simulink model "Proposed_converter"  (R2023b)
settings: Solver=VariableStepAuto  StartTime=0.0  StopTime=30e-3  RelTol=1e-3
undefined symbols (not defined in the file): pro
libraries: spsVoltageMeasurementLib x22, spsCurrentMeasurementLib x21, spsSeriesRLCBranchLib x17, spsDiodeLib x11, spsIdealSwitchLib x6, spsDCVoltageSourceLib x2, spspowerguiLib x2
settings Model: Creator=JesperBertelsen  LastModifiedBy=JesperBertelsen

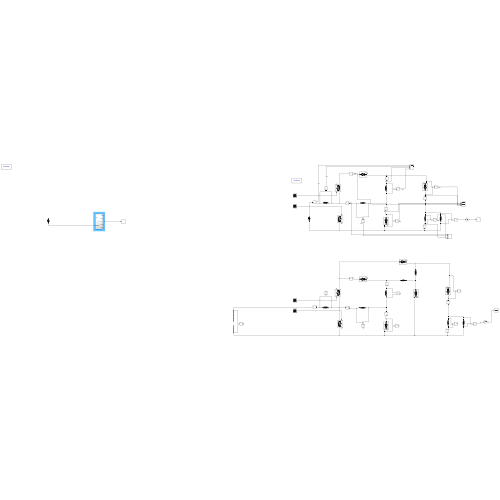
[thumbnail: Simulink's stored preview of the top-level diagram]
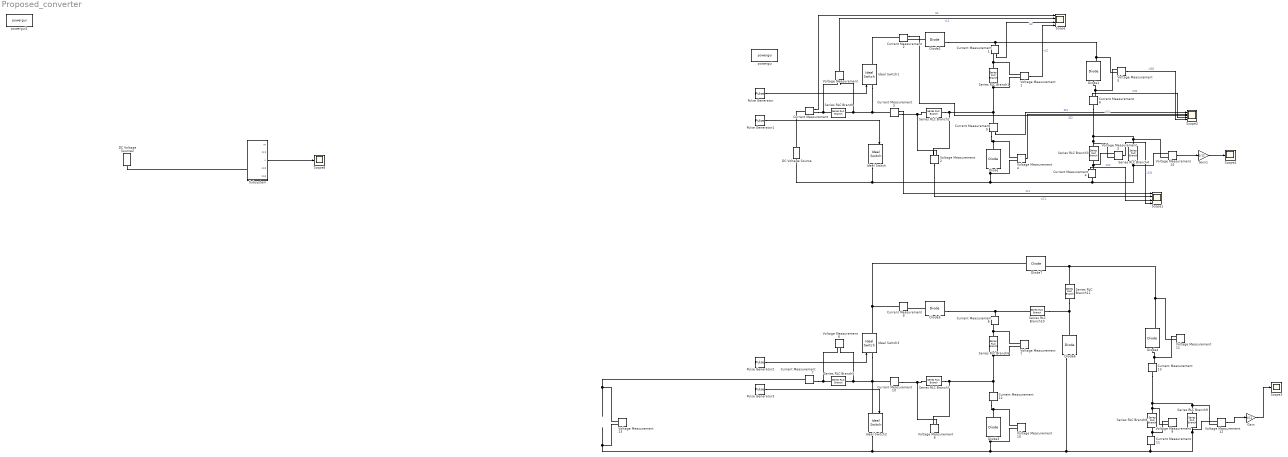
== system Proposed_converter ==
  Current Measurement{,1..13} (14 alike) : spsCurrentMeasurementLib/Current Measurement  PhasorSimulation=off  OutputType=Complex  PSBequivalent=0
  DC Voltage Source : spsDCVoltageSourceLib/DC Voltage Source  Amplitude=pro.Vi  Measurements=None
  DC Voltage Source2 : spsDCVoltageSourceLib/DC Voltage Source  Amplitude=pro.Vi  Measurements=None
  Diode{,1..7} (8 alike) : spsDiodeLib/Diode  Ron=pro.rD  Lon=0  Vf=0.8  IC=0  UseSnubber=0  Rs=0  Cs=0  Measurements=on
  Gain : Gain  Gain=1/12
  Gain1 : Gain  Gain=1/12
  Ideal Switch{,1..3} (4 alike) : spsIdealSwitchLib/Ideal Switch  Ron=0.001  Lon=0  IC=0  Rs=1e5  Cs=inf  Measurements=on
  Pulse Generator{,1..3} (4 alike) : DiscretePulseGenerator  PulseType=Time based  Period=1/pro.f  PulseWidth=50
  Scope : Scope  NumInputPorts=4
  Scope1 : Scope  NumInputPorts=4
  Scope2 : Scope  NumInputPorts=5
  Scope3 : Scope
  Scope4 : Scope
  Scope8 : Scope
  Series RLC Branch : spsSeriesRLCBranchLib/Series RLC Branch  LConnTagsString=__new0  RConnTagsString=__new0  BranchType=L  Resistance=1  Inductance=pro.L1  SetiL0=off  InitialCurrent=0  Capacitance=1e-6  Setx0=off  InitialVoltage=0  Measurements=Branch voltage and current
  Series RLC Branch1 : spsSeriesRLCBranchLib/Series RLC Branch  LConnTagsString=__new0  RConnTagsString=__new0  BranchType=L  Resistance=1  Inductance=pro.L2  SetiL0=off  InitialCurrent=0  Capacitance=1e-6  Setx0=off  InitialVoltage=0  Measurements=Branch voltage and current
  Series RLC Branch10 : spsSeriesRLCBranchLib/Series RLC Branch  LConnTagsString=__new0  RConnTagsString=__new0  BranchType=C  Resistance=1  Inductance=1e-3  SetiL0=off  InitialCurrent=0  Capacitance=pro.C1  Setx0=off  InitialVoltage=0  Measurements=Branch voltage and current
  Series RLC Branch11 : spsSeriesRLCBranchLib/Series RLC Branch  LConnTagsString=__new0  RConnTagsString=__new0  BranchType=L  Resistance=1  Inductance=pro.L2  SetiL0=off  InitialCurrent=0  Capacitance=1e-6  Setx0=off  InitialVoltage=0  Measurements=Branch voltage and current
  Series RLC Branch2 : spsSeriesRLCBranchLib/Series RLC Branch  LConnTagsString=__new0  RConnTagsString=__new0  BranchType=C  Resistance=1  Inductance=1e-3  SetiL0=off  InitialCurrent=0  Capacitance=pro.C1  Setx0=off  InitialVoltage=0  Measurements=Branch voltage and current
  Series RLC Branch3 : spsSeriesRLCBranchLib/Series RLC Branch  LConnTagsString=__new0  RConnTagsString=__new0  BranchType=C  Resistance=1  Inductance=1e-3  SetiL0=off  InitialCurrent=0  Capacitance=pro.C1  Setx0=off  InitialVoltage=0  Measurements=None
  Series RLC Branch4 : spsSeriesRLCBranchLib/Series RLC Branch  LConnTagsString=__new0  RConnTagsString=__new0  BranchType=R  Resistance=pro.R  Inductance=pro.L1  SetiL0=off  InitialCurrent=0  Capacitance=1e-6  Setx0=off  InitialVoltage=0  Measurements=None
  Series RLC Branch5 : spsSeriesRLCBranchLib/Series RLC Branch  LConnTagsString=__new0  RConnTagsString=__new0  BranchType=L  Resistance=1  Inductance=pro.L1  SetiL0=off  InitialCurrent=0  Capacitance=1e-6  Setx0=off  InitialVoltage=0  Measurements=Branch voltage and current
  Series RLC Branch6 : spsSeriesRLCBranchLib/Series RLC Branch  LConnTagsString=__new0  RConnTagsString=__new0  BranchType=L  Resistance=1  Inductance=pro.L2  SetiL0=off  InitialCurrent=0  Capacitance=1e-6  Setx0=off  InitialVoltage=0  Measurements=Branch voltage and current
  Series RLC Branch7 : spsSeriesRLCBranchLib/Series RLC Branch  LConnTagsString=__new0  RConnTagsString=__new0  BranchType=C  Resistance=1  Inductance=1e-3  SetiL0=off  InitialCurrent=0  Capacitance=pro.C1  Setx0=off  InitialVoltage=0  Measurements=Branch voltage and current
  Series RLC Branch8 : spsSeriesRLCBranchLib/Series RLC Branch  LConnTagsString=__new0  RConnTagsString=__new0  BranchType=C  Resistance=1  Inductance=1e-3  SetiL0=off  InitialCurrent=0  Capacitance=pro.C1  Setx0=off  InitialVoltage=0  Measurements=None
  Series RLC Branch9 : spsSeriesRLCBranchLib/Series RLC Branch  LConnTagsString=__new0  RConnTagsString=__new0  BranchType=R  Resistance=pro.R  Inductance=pro.L1  SetiL0=off  InitialCurrent=0  Capacitance=1e-6  Setx0=off  InitialVoltage=0  Measurements=None
  Subsystem : Subsystem
  Voltage Measurement{,1..14} (15 alike) : spsVoltageMeasurementLib/Voltage Measurement  PhasorSimulation=off  OutputType=Complex  PSBequivalent=0
  powergui : spspowerguiLib/powergui  Priority=1  SimulationMode=Continuous  SampleTime=50e-6  frequency=60  Iterations=50  frequencyindice=0  Pbase=100e6  ErrMax=1e-4  UnitsV=kV  UnitsW=MW  buscounter=0  FunctionMessages=off  echomessages=off  EnableUseOfTLC=off  CurrentSourceSwitches=off  DisableSnubberDevices=off  DisableRonSwitches=off  DisableVfSwitches=off  DisplayEquations=off  AutomaticDiscreteSolvers=off  SolverType=Tustin/Backward Euler (TBE)  Interpol=off  ExternalGateDelay=off  methode=off  Ts=100  x0status=blocks  SPID=on  SwTol=0  HookPort=off  NonlinearTolerance=1e-4  nMaxIteration=100  ContinueOnMaxIteration=off  RestoreLinks=warning  ResistiveCurrentMeasurement=off  Frange=[0:2:500]  Ylog=off  Xlog=on  ShowGrid=off  save=off  variable=ZData  structure=0  ZoomFFT=off  StartTime=0.0  cycles=1  DisplayStyle=1  fundamental=60  FreqAxis=off  MaxFrequency=1000  frequencyindicesteady=1  RmsSteady=1  display=off
  powergui1 : spspowerguiLib/powergui  Priority=1  SimulationMode=Continuous  SampleTime=50e-6  frequency=60  Iterations=50  frequencyindice=0  Pbase=100e6  ErrMax=1e-4  UnitsV=kV  UnitsW=MW  buscounter=0  FunctionMessages=off  echomessages=off  EnableUseOfTLC=off  CurrentSourceSwitches=off  DisableSnubberDevices=off  DisableRonSwitches=off  DisableVfSwitches=off  DisplayEquations=off  AutomaticDiscreteSolvers=off  SolverType=Tustin/Backward Euler (TBE)  Interpol=off  ExternalGateDelay=off  methode=off  Ts=100  x0status=blocks  SPID=on  SwTol=0  HookPort=off  NonlinearTolerance=1e-4  nMaxIteration=100  ContinueOnMaxIteration=off  RestoreLinks=warning  ResistiveCurrentMeasurement=off  Frange=[0:2:500]  Ylog=off  Xlog=on  ShowGrid=off  save=off  variable=ZData  structure=0  ZoomFFT=off  StartTime=0.0  cycles=1  DisplayStyle=1  fundamental=60  FreqAxis=off  MaxFrequency=1000  frequencyindicesteady=1  RmsSteady=1  display=off
  wires:
  Pulse Generator/1 -> Ideal Switch1/1
  Pulse Generator1/1 -> Ideal Switch/1
  Current Measurement/1 -> Scope/1  "iL1"
  Voltage Measurement/1 -> Scope/2  "vL1"
  Voltage Measurement1/1 -> Scope/4  "vL2"
  Current Measurement1/1 -> Scope/3  "iL2"
  Voltage Measurement2/1 -> Scope1/2  "vC1"
  Current Measurement3/1 -> Scope1/1  "iC1"
  Voltage Measurement3/1 -> Scope1/4  "vCO"
  Current Measurement4/1 -> Scope1/3  "iCO"
  Voltage Measurement4/1 -> Scope2/2  "vD1"
  Current Measurement5/1 -> Scope2/1  "iD1"
  Voltage Measurement5/1 -> Scope2/5  "vDO"
  Current Measurement6/1 -> Scope2/4  "iCO"
  Current Measurement2/1 -> Scope2/3  "iD2"
  Pulse Generator2/1 -> Ideal Switch3/1
  Pulse Generator3/1 -> Ideal Switch2/1
  Voltage Measurement12/1 -> Gain/1
  Gain/1 -> Scope3/1
  Voltage Measurement14/1 -> Gain1/1
  Gain1/1 -> Scope4/1
  Subsystem/3(v) -> Scope8/1
  connections:
  Series RLC Branch/LConn1 -- Current Measurement/RConn1 -- Voltage Measurement/LConn1
  Ideal Switch1/LConn1 -- Current Measurement3/LConn1 -- Series RLC Branch/RConn1 -- Voltage Measurement/LConn2
  Series RLC Branch2/RConn1 -- Voltage Measurement2/LConn2 -- Voltage Measurement1/LConn2 -- Series RLC Branch1/RConn1 -- Current Measurement5/LConn1
  DC Voltage Source/LConn1 -- Ideal Switch/RConn1 -- Voltage Measurement4/LConn2 -- Diode/RConn1 -- Current Measurement4/LConn1 -- Voltage Measurement14/LConn1 -- Series RLC Branch4/LConn1
  Diode2/RConn1 -- Current Measurement1/LConn1 -- Voltage Measurement5/LConn2 -- Diode1/RConn1
  Series RLC Branch3/RConn1 -- Voltage Measurement3/LConn2 -- Voltage Measurement14/LConn2 -- Series RLC Branch4/RConn1 -- Current Measurement6/LConn1
  Current Measurement/LConn1 -- DC Voltage Source/RConn1
  Series RLC Branch1/LConn1 -- Voltage Measurement1/LConn1 -- Current Measurement1/RConn1
  Current Measurement2/LConn1 -- Ideal Switch1/RConn1
  Diode2/LConn1 -- Current Measurement2/RConn1
  Series RLC Branch2/LConn1 -- Current Measurement3/RConn1 -- Voltage Measurement2/LConn1
  Voltage Measurement3/LConn1 -- Current Measurement4/RConn1 -- Series RLC Branch3/LConn1
  Current Measurement5/RConn1 -- Diode/LConn1 -- Voltage Measurement4/LConn1
  Voltage Measurement5/LConn1 -- Diode1/LConn1 -- Current Measurement6/RConn1
  Diode6/RConn1 -- Voltage Measurement10/LConn2 -- Diode3/RConn1 -- Voltage Measurement13/LConn2 -- Ideal Switch2/RConn1 -- Current Measurement11/LConn1 -- Voltage Measurement12/LConn1 -- Series RLC Branch9/LConn1
  Series RLC Branch6/LConn1 -- Voltage Measurement7/LConn1 -- Current Measurement8/RConn1
  Voltage Measurement11/LConn1 -- Current Measurement13/RConn1 -- Diode4/LConn1
  Series RLC Branch8/RConn1 -- Voltage Measurement9/LConn2 -- Voltage Measurement12/LConn2 -- Series RLC Branch9/RConn1 -- Current Measurement13/LConn1
  Diode6/LConn1 -- Series RLC Branch11/RConn1 -- Series RLC Branch10/RConn1
  Voltage Measurement10/LConn1 -- Diode3/LConn1 -- Current Measurement12/RConn1
  Series RLC Branch7/RConn1 -- Voltage Measurement8/LConn2 -- Voltage Measurement7/LConn2 -- Series RLC Branch6/RConn1 -- Current Measurement12/LConn1
  Ideal Switch2/LConn1 -- Series RLC Branch5/RConn1 -- Voltage Measurement6/LConn2 -- Current Measurement10/LConn1 -- Ideal Switch3/LConn1
  Voltage Measurement9/LConn1 -- Current Measurement11/RConn1 -- Series RLC Branch8/LConn1
  Series RLC Branch7/LConn1 -- Current Measurement10/RConn1 -- Voltage Measurement8/LConn1
  Voltage Measurement6/LConn1 -- Series RLC Branch5/LConn1 -- Current Measurement7/RConn1
  Voltage Measurement13/LConn1 -- Current Measurement7/LConn1
  Current Measurement9/LConn1 -- Diode7/LConn1 -- Ideal Switch3/RConn1
  Diode5/RConn1 -- Series RLC Branch10/LConn1 -- Current Measurement8/LConn1
  Diode5/LConn1 -- Current Measurement9/RConn1
  Diode4/RConn1 -- Voltage Measurement11/LConn2 -- Series RLC Branch11/LConn1 -- Diode7/RConn1
  DC Voltage Source2/LConn1 -- Subsystem/LConn2

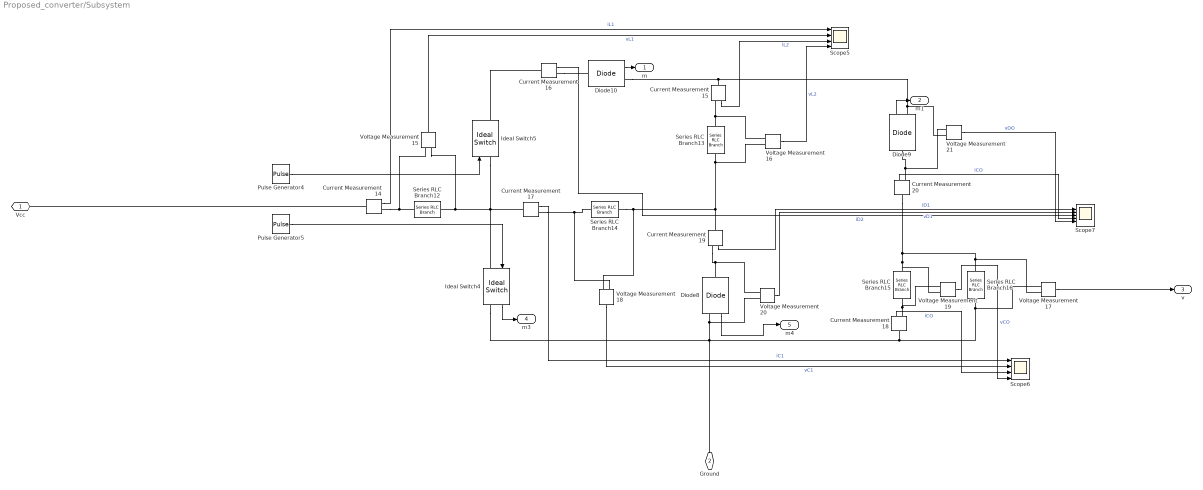
== system Proposed_converter/Subsystem ==
  Current Measurement{14..20} (7 alike) : spsCurrentMeasurementLib/Current Measurement  PhasorSimulation=off  OutputType=Complex  PSBequivalent=0
  Diode10 : spsDiodeLib/Diode  Ron=pro.rD  Lon=0  Vf=0.8  IC=0  UseSnubber=0  Rs=0  Cs=0  Measurements=on
  Diode8 : spsDiodeLib/Diode  Ron=pro.rD  Lon=0  Vf=0.8  IC=0  UseSnubber=0  Rs=0  Cs=0  Measurements=on
  Diode9 : spsDiodeLib/Diode  Ron=pro.rD  Lon=0  Vf=0.8  IC=0  UseSnubber=0  Rs=0  Cs=0  Measurements=on
  Ideal Switch4 : spsIdealSwitchLib/Ideal Switch  Ron=0.001  Lon=0  IC=0  Rs=1e5  Cs=inf  Measurements=on
  Ideal Switch5 : spsIdealSwitchLib/Ideal Switch  Ron=0.001  Lon=0  IC=0  Rs=1e5  Cs=inf  Measurements=on
  Pulse Generator4 : DiscretePulseGenerator  PulseType=Time based  Period=1/pro.f  PulseWidth=50
  Pulse Generator5 : DiscretePulseGenerator  PulseType=Time based  Period=1/pro.f  PulseWidth=50
  Scope5 : Scope  NumInputPorts=4
  Scope6 : Scope  NumInputPorts=4
  Scope7 : Scope  NumInputPorts=5
  Series RLC Branch12 : spsSeriesRLCBranchLib/Series RLC Branch  LConnTagsString=__new0  RConnTagsString=__new0  BranchType=L  Resistance=1  Inductance=pro.L1  SetiL0=off  InitialCurrent=0  Capacitance=1e-6  Setx0=off  InitialVoltage=0  Measurements=Branch voltage and current
  Series RLC Branch13 : spsSeriesRLCBranchLib/Series RLC Branch  LConnTagsString=__new0  RConnTagsString=__new0  BranchType=L  Resistance=1  Inductance=pro.L2  SetiL0=off  InitialCurrent=0  Capacitance=1e-6  Setx0=off  InitialVoltage=0  Measurements=Branch voltage and current
  Series RLC Branch14 : spsSeriesRLCBranchLib/Series RLC Branch  LConnTagsString=__new0  RConnTagsString=__new0  BranchType=C  Resistance=1  Inductance=1e-3  SetiL0=off  InitialCurrent=0  Capacitance=pro.C1  Setx0=off  InitialVoltage=0  Measurements=Branch voltage and current
  Series RLC Branch15 : spsSeriesRLCBranchLib/Series RLC Branch  LConnTagsString=__new0  RConnTagsString=__new0  BranchType=C  Resistance=1  Inductance=1e-3  SetiL0=off  InitialCurrent=0  Capacitance=pro.C1  Setx0=off  InitialVoltage=0  Measurements=None
  Series RLC Branch16 : spsSeriesRLCBranchLib/Series RLC Branch  LConnTagsString=__new0  RConnTagsString=__new0  BranchType=R  Resistance=pro.R  Inductance=pro.L1  SetiL0=off  InitialCurrent=0  Capacitance=1e-6  Setx0=off  InitialVoltage=0  Measurements=None
  Voltage Measurement{15..21} (7 alike) : spsVoltageMeasurementLib/Voltage Measurement  PhasorSimulation=off  OutputType=Complex  PSBequivalent=0
  Vcc : PMIOPort  Side=Left
  Ground : PMIOPort  Port=2  Side=Left
  m : Outport
  m1 : Outport  Port=2
  v : Outport  Port=3
  m3 : Outport  Port=4
  m4 : Outport  Port=5
  wires:
  Diode10/1 -> m/1
  Current Measurement19/1 -> Scope7/1  "iD1"
  Diode8/1 -> m4/1
  Voltage Measurement15/1 -> Scope5/2  "vL1"
  Voltage Measurement19/1 -> Scope6/4  "vCO"
  Current Measurement17/1 -> Scope6/1  "iC1"
  Pulse Generator5/1 -> Ideal Switch4/1
  Current Measurement18/1 -> Scope6/3  "iCO"
  Voltage Measurement21/1 -> Scope7/5  "vDO"
  Voltage Measurement17/1 -> v/1
  Current Measurement15/1 -> Scope5/3  "iL2"
  Voltage Measurement20/1 -> Scope7/2  "vD1"
  Voltage Measurement16/1 -> Scope5/4  "vL2"
  Current Measurement14/1 -> Scope5/1  "iL1"
  Pulse Generator4/1 -> Ideal Switch5/1
  Ideal Switch4/1 -> m3/1
  Voltage Measurement18/1 -> Scope6/2  "vC1"
  Diode9/1 -> m1/1
  Current Measurement16/1 -> Scope7/3  "iD2"
  Current Measurement20/1 -> Scope7/4  "iCO"
  connections:
  Current Measurement14/LConn1 -- Vcc/RConn1
  Voltage Measurement20/LConn1 -- Current Measurement19/RConn1 -- Diode8/LConn1
  Current Measurement20/RConn1 -- Voltage Measurement21/LConn1 -- Diode9/LConn1
  Voltage Measurement18/LConn1 -- Series RLC Branch14/LConn1 -- Current Measurement17/RConn1
  Current Measurement19/LConn1 -- Voltage Measurement16/LConn2 -- Series RLC Branch13/RConn1 -- Series RLC Branch14/RConn1 -- Voltage Measurement18/LConn2
  Ideal Switch5/RConn1 -- Current Measurement16/LConn1
  Series RLC Branch15/LConn1 -- Voltage Measurement19/LConn1 -- Current Measurement18/RConn1
  Voltage Measurement15/LConn2 -- Ideal Switch4/LConn1 -- Ideal Switch5/LConn1 -- Current Measurement17/LConn1 -- Series RLC Branch12/RConn1
  Series RLC Branch16/LConn1 -- Voltage Measurement17/LConn1 -- Ground/RConn1 -- Ideal Switch4/RConn1 -- Voltage Measurement20/LConn2 -- Diode8/RConn1 -- Current Measurement18/LConn1
  Current Measurement15/RConn1 -- Series RLC Branch13/LConn1 -- Voltage Measurement16/LConn1
  Diode9/RConn1 -- Voltage Measurement21/LConn2 -- Diode10/RConn1 -- Current Measurement15/LConn1
  Current Measurement20/LConn1 -- Voltage Measurement17/LConn2 -- Series RLC Branch16/RConn1 -- Series RLC Branch15/RConn1 -- Voltage Measurement19/LConn2
  Voltage Measurement15/LConn1 -- Series RLC Branch12/LConn1 -- Current Measurement14/RConn1
  Current Measurement16/RConn1 -- Diode10/LConn1
